simulink model "Car_23_Jan_test_2012b"  (R2012b)
settings: Solver=ode5  StartTime=0.0  StopTime=inf  FixedStep=sample_time  RelTol=1e-3
InitFcn:
  | sample_time=0.005;%0.004;%0.0025;%0.02;
  | sample_time_Vicon = 0.005;
  | DeltaT = 0.02;
  | g = 9.81;
  | H0 = g%0.3165;
  | Kl = 1;
  | 
  | Q6_mass = 0.84;
  | 
  | Q6_Omega_r = 1.5; %for horizon ref
  | Q6_Zeta_r = 0.5; %for horizon ref
  | Q6_Omega_r_h = 2;%for vertical ref
  | Q6_Zeta_r_h = 2; %for vertical ref
  | 
  | 
  | Q6_Omega = 1.5; %for horizon control
  | Q6_Zeta = 0.5; %for horizon control
  | Q6_Omega_h= 2; %for vertical control
  | Q6_Zeta_h = 0.7; %for vertical control
  | 
  | 
  | Q6_acc_max = 5;%horizontal max acc
  | Q6_acc_max_h = 3;%horizontal max acc
  | 
  | omega_circle = 72*pi/180;
  | omega_h = 0.1;%Ascending speed
  | PI = pi;
  | Circle_R = 2.5;
  | MAX_Height = -2;
undefined symbols (not defined in the file): DiscIntNeverNeededParam
libraries: X330_Control x5, dspswit3 x5, simulink x4
(part 2 of 2)

== matlab function Car_23_Jan_test_2012b/UAV 1/Trajectory Logic/trackbounded ==
  data: cpx input; cpy input; region output; cvx input; cvy input; newx output; newy output; newregion output; estsecond input; chkfinalx output; chkfinaly output; chknum output; directionflag output; distanceall output; limitspeed input
function [region,newx,newy,newregion,chkfinalx,chkfinaly,chknum,directionflag,distanceall]  = fcn(cpx,cpy,cvx,cvy,estsecond,limitspeed)
%#codegen
%cp = [cpy,cpx,0];
%cpest = [estrawy, estrawx,0];
%%database of check points
chk0x = -0.7975;
chk0y = 1.469;
chk1x = -1.008;
chk1y = 0.4326;
chk2x = -1.068;
chk2y = -0.6832;
chk3x = -0.5072;
chk3y = -1.342;
chk4x = 0.4105;
chk4y = -1.356;
chk5x = 1.225;
chk5y = -1.322;
chk6x = 1.733;
chk6y = -0.7022;
chk7x = 1.446;
chk7y = 0.6614;
chk8x = 1.136;
chk8y = 1.384;
chk9x = 0.3114;
chk9y = 1.798;
%%%%%%%%%%%%%%%%%%%%%%%%%%%%%%%%%%%%%%%%%%%%%%%%%%%%%%%%%%%
chk0 = [chk0y,chk0x,0];
chk1 = [chk1y,chk1x,0];
chk2 = [chk2y,chk2x,0];
chk3 = [chk3y,chk3x,0];
chk4 = [chk4y,chk4x,0];
chk5 = [chk5y,chk5x,0];
distance01 = sqrt((chk0y-chk1y)^2+(chk0x-chk1x)^2);
distance12 = sqrt((chk2y-chk1y)^2+(chk2x-chk1x)^2);
distance23 = sqrt((chk2y-chk3y)^2+(chk2x-chk3x)^2);
distance34 = sqrt((chk3y-chk4y)^2+(chk3x-chk4x)^2);
distance45 = sqrt((chk4y-chk5y)^2+(chk4x-chk5x)^2);
distance56 = sqrt((chk5y-chk6y)^2+(chk5x-chk6x)^2);
distance67 = sqrt((chk6y-chk7y)^2+(chk6x-chk7x)^2);
distance78 = sqrt((chk7y-chk8y)^2+(chk7x-chk8x)^2);
distance89 = sqrt((chk8y-chk9y)^2+(chk8x-chk9x)^2);
distance90 = sqrt((chk9y-chk0y)^2+(chk9x-chk0x)^2);
distanceall = distance01 + distance12 + distance23+distance34+distance45+distance56+distance67+distance78+distance89+distance90;
%%%%%%%%%%%%%%%%%%%%%%%%%%%%%%%%%%%%%%%%%%%%%%%%%%%%%%%%%%%%%%%%%%%%%%%%%%%%%%%%%%%%%%region selector
if(cpx>-2 && cpx<=-1 && cpy>1 && cpy<=2)
    region = 0;
elseif(cpx>-1 && cpx<=0 && cpy>1 && cpy<=2 )
    region = 1;
elseif(cpx>0 && cpx<=1 && cpy>1 && cpy<=2 )
    region = 2;
elseif(cpx>-2 && cpx<=-1 && cpy>0 &&cpy<=1)
    region = 3;
elseif(cpx>-1 && cpx<=0 && cpy>0 && cpy<=1)
    region = 4;
elseif(cpx>-2 && cpx<=-1 &&cpy>-1 && cpy<=0)
    region = 5;
elseif(cpx>-1 && cpx<=0 && cpy>-1 && cpy<=0)
    region = 6;
elseif(cpx>-2 && cpx<=-1 && cpy>-2 && cpy<=-1)
    region = 7;
elseif(cpx>-1 && cpx<=0 && cpy>-2 && cpy<=-1)
    region = 8;
elseif(cpx>0 && cpx<=1 && cpy>-2 && cpy<=-1)
    region = 9;
elseif(cpx>1 && cpx<=2 && cpy>-2 && cpy<=-1)
    region = 10;
elseif(cpx>0 && cpx<=1 && cpy>-1 && cpy<=0)
    region = 11;
elseif(cpx>1 && cpx<=2 && cpy>-1 && cpy<=0)
    region = 12;
elseif(cpx>1 && cpx<=2 && cpy>0 && cpy<=1)
    region = 13;
elseif(cpx>1 && cpx<=2 && cpy>1 && cpy<=2)
    region = 14;
elseif(cpx>0 && cpx<=1 && cpy>0 && cpy<=1)
    region = 15;
elseif(cpx>2 && cpx<=3 && cpy>-2 && cpy<=-1)
    region = 16;
elseif(cpx>1 && cpx<=2 && cpy>-3 && cpy<=-2)
    region = 17;
elseif(cpx>2 && cpx<=3 && cpy>-3 && cpy<=-2)
    region = 18;
elseif(cpx>0 && cpx<=1 && cpy>-3 && cpy<=-2)
    region = 19;
elseif(cpx>-1 && cpx<=0 && cpy>-3 && cpy<=-2)
    region = 20;
elseif(cpx>2 && cpx<=3 && cpy>-1 && cpy<=0)
    region = 21;
elseif(cpx>2 && cpx<=3 && cpy>0 && cpy<=1)
    region = 22;
elseif(cpx>1 && cpx<=2 && cpy>2 && cpy<=3)
    region = 23;
elseif(cpx>0 && cpx<=1 && cpy>2 && cpy<=3)
    region = 24;
elseif(cpx>-1 && cpx<=0 && cpy>2 && cpy<=3)
    region = 25;
else
    region = -1;
end
%%%%%%%%%%%%%%%%%%%%%%%%%%%%%%%%%%%%%%%%%%%%%%%%%%%%%%%%%%%%%%%%%%%%%%%%%%%%%%%%%%%%%%%%%%%%%%%%%%
if(region == 0 ||region==3||region==4)
    %%%%%%%%%%%%%%%%calculate point to line distance%%%%%%%%%%%
    %a = chk1 - chk0;
   % b = cp - chk0;
    %d = norm(cross(a,b)) / norm(a);
    angle = atan2((chk1x-chk0x),(chk1y-chk0y));
    samplex = chk0x;
    sampley = chk0y;
    zero = 1;

elseif(region == 5||region==6)
    %a = chk2 - chk1;
   % b = cp - chk1;
   % d = norm(cross(a,b)) / norm(a);
    angle = atan2((chk2x-chk1x),(chk2y-chk1y));
    zero = 1;
    samplex = chk1x;
    sampley = chk1y;
elseif(region == 7||region==8)
    %a = chk3 - chk2;
    %b = cp - chk2;
   % d = norm(cross(a,b)) / norm(a);
    angle = atan2((chk3x-chk2x),(chk3y-chk2y));
    zero = 1;
    samplex = chk2x;
    sampley = chk2y;
elseif(region == 9 || region==11||region==19||region==20)
   % a = chk4 - chk3;
   % b = cp - chk3;
    %d = norm(cross(a,b)) / norm(a);
    angle = atan2((chk4x-chk3x),(chk4y-chk3y));
    zero = 1;
      samplex = chk3x;
    sampley = chk3y;
elseif(region == 10 || region==17||region==18)
    %a = chk5 - chk4;
    %b = cp - chk4;
    %d = norm(cross(a,b)) / norm(a);
    angle = atan2((chk5x-chk4x),(chk5y-chk4y));
    zero = 1;
    samplex = chk4x;
    sampley = chk4y;
elseif(region == 12 || region==16||region==21)
    %a = chk6 - chk5;
    %b = cp - chk5;
    %d = norm(cross(a,b)) / norm(a);
    angle = atan2((chk6x-chk5x),(chk6y-chk5y));
    zero = 1;
    samplex = chk5x;
    sampley = chk5y;
elseif(region == 22 || region==13)
    %a = chk7 - chk6;
    %b = cp - chk6;
    %d = norm(cross(a,b)) / norm(a);
    angle = atan2((chk7x-chk6x),(chk7y-chk6y));
    zero = 1;
    samplex = chk6x;
    sampley = chk6y;
elseif(region == 14)
    %a = chk8 - chk7;
    %b = cp - chk7;
    %d = norm(cross(a,b)) / norm(a);
    angle = atan2((chk8x-chk7x),(chk8y-chk7y));
    zero = 1;
    samplex = chk7x;
    sampley = chk7y;
elseif(region == 2||region==23||region==24)
    %a = chk9 - chk8;
    %b = cp - chk8;
    %d = norm(cross(a,b)) / norm(a);
    angle = atan2((chk9x-chk8x),(chk9y-chk8y));
    zero = 1;
    samplex = chk8x;
    sampley = chk8y;
elseif(region == 25||region==1)
    %a = chk0 - chk9;
    %b = cp - chk9;
    %d = norm(cross(a,b)) / norm(a);
    angle = atan2((chk0x-chk9x),(chk0y-chk9y));
    zero = 1;
    samplex = chk9x;
    sampley = chk9y;
else
    %a = -1;
   % b = -1;
    %d = -1;
    angle = -1;%%% i know this is not correct i will add one more zero coefficient to cancel this case
    zero = 0;
    samplex = 0;
    sampley = 0;
end


%%%%%%%%%%%%%%%%%%%%%%%%%%%%%%%%%%%%%%%%%%%%%%%%%%%%%%%%%%%%%%%%%%%%%%%%%%%%%%%%%%%%%%%%%%%%%%%%%%
% %%calculate project point on the check point line
if(zero == 0)%%if out of boundary none of the region match
        newy = 100;
        newx = 100;
else   %%match the region

        if(angle == 0 ||angle == 180)
            newx  = samplex;
            newy = cpy;
        elseif(angle == 90 || angle == 270)
            newx = cpx;
            newy = sampley;
        else
         kk = -1/(tan(angle));
         m = cpx - kk*cpy ;
         k = tan(angle);
         newy = (samplex - k*sampley - m)/(kk - k);
         newx = kk*newy + m;
         end

end

if(newx>-2 && newx<=-1 && newy>1 && newy<=2)
    newregion = 0;
elseif(newx>-1 && newx<=0 && newy>1 && newy<=2 )
    newregion = 1;
elseif(newx>0 && newx<=1 && newy>1 && newy<=2 )
    newregion = 2;
elseif(newx>-2 && newx<=-1 && newy>0 &&newy<=1)
    newregion = 3;
elseif(newx>-1 && newx<=0 && newy>0 && newy<=1)
    newregion = 4;
elseif(newx>-2 && newx<=-1 &&newy>-1 && newy<=0)
    newregion = 5;
elseif(newx>-1 && newx<=0 && newy>-1 && newy<=0)
    newregion = 6;
elseif(newx>-2 && newx<=-1 && newy>-2 && newy<=-1)
    newregion = 7;
elseif(newx>-1 && newx<=0 && newy>-2 && newy<=-1)
    newregion = 8;
elseif(newx>0 && newx<=1 && newy>-2 && newy<=-1)
    newregion = 9;
elseif(newx>1 && newx<=2 && newy>-2 && newy<=-1)
    newregion = 10;
elseif(newx>0 && newx<=1 && newy>-1 && newy<=0)
    newregion = 11;
elseif(newx>1 && newx<=2 && newy>-1 && newy<=0)
    newregion = 12;
elseif(newx>1 && newx<=2 && newy>0 && newy<=1)
    newregion = 13;
elseif(newx>1 && newx<=2 && newy>1 && newy<=2)
    newregion = 14;
elseif(newx>0 && newx<=1 && newy>0 && newy<=1)
    newregion = 15;
elseif(newx>2 && newx<=3 && newy>-2 && newy<=-1)
    newregion = 16;
elseif(newx>1 && newx<=2 && newy>-3 && newy<=-2)
    newregion = 17;
elseif(newx>2 && newx<=3 && newy>-3 && newy<=-2)
    newregion = 18;
elseif(newx>0 && newx<=1 && newy>-3 && newy<=-2)
    newregion = 19;
elseif(newx>-1 && newx<=0 && newy>-3 && newy<=-2)
    newregion = 20;
elseif(newx>2 && newx<=3 && newy>-1 && newy<=0)
    newregion = 21;
elseif(newx>2 && newx<=3 && newy>0 && newy<=1)
    newregion = 22;
elseif(newx>1 && newx<=2 && newy>2 && newy<=3)
    newregion = 23;
elseif(newx>0 && newx<=1 && newy>2 && newy<=3)
    newregion = 24;
elseif(newx>-1 && newx<=0 && newy>2 && newy<=3)
    newregion = 25;
else
    newregion = -1;
end

%%%%%%%%%%%%%%%%%%%%%%%%%%%%%%%%%%%%%%%%%%%%%%%%%%%%%%%%%%%%%%%%%%%%%%%%%%%%
% if(posx>-2 && posx<=-1 && posy>1 && posy<=2)
%     posregion = 0;
% elseif(posx>-1 && posx<=0 && posy>1 && posy<=2 )
%     posregion = 1;
% elseif(posx>0 && posx<=1 && posy>1 && posy<=2 )
%     posregion = 2;
% elseif(posx>-2 && posx<=-1 && posy>0 &&posy<=1)
%     posregion = 3;
% elseif(posx>-1 && posx<=0 && posy>0 && posy<=1)
%     posregion = 4;
% elseif(posx>-2 && posx<=-1 &&posy>-1 && posy<=0)
%     posregion = 5;
% elseif(posx>-1 && posx<=0 && posy>-1 && posy<=0)
%     posregion = 6;
% elseif(posx>-2 && posx<=-1 && posy>-2 && posy<=-1)
%     posregion = 7;
% elseif(posx>-1 && posx<=0 && posy>-2 && posy<=-1)
%     posregion = 8;
% elseif(posx>0 && posx<=1 && posy>-2 && posy<=-1)
%     posregion = 9;
% elseif(posx>1 && posx<=2 && posy>-2 && posy<=-1)
%     posregion = 10;
% elseif(posx>0 && posx<=1 && posy>-1 && posy<=0)
%     posregion = 11;
% elseif(posx>1 && posx<=2 && posy>-1 && posy<=0)
%     posregion = 12;
% elseif(posx>1 && posx<=2 && posy>0 && posy<=1)
%     posregion = 13;
% elseif(posx>1 && posx<=2 && posy>1 && posy<=2)
%     posregion = 14;
% elseif(posx>0 && posx<=1 && posy>0 && posy<=1)
%     posregion = 15;
% elseif(posx>2 && posx<=3 && posy>-2 && posy<=-1)
%     posregion = 16;
% elseif(posx>1 && posx<=2 && posy>-3 && posy<=-2)
%     posregion = 17;
% elseif(posx>2 && posx<=3 && posy>-3 && posy<=-2)
%     posregion = 18;
% elseif(posx>0 && posx<=1 && posy>-3 && posy<=-2)
%     posregion = 19;
% elseif(posx>-1 && posx<=0 && posy>-3 && posy<=-2)
%     posregion = 20;
% elseif(posx>2 && posx<=3 && posy>-1 && posy<=0)
%     posregion = 21;
% elseif(posx>2 && posx<=3 && posy>0 && posy<=1)
%     posregion = 22;
% elseif(posx>1 && posx<=2 && posy>2 && posy<=3)
%     posregion = 23;
% elseif(posx>0 && posx<=1 && posy>2 && posy<=3)
%    posregion = 24;
% elseif(posx>-1 && posx<=0 && posy>2 && posy<=3)
%     posregion = 25;
% else
%     posregion = -1;
% end


%%%%%%%%%%%%%%%%%%%%%%%%%%%%%%%%%%%%%%%%%%%%%%%%%%%%%%%%%%%%%%%%%%%%%%%%%
velangle = atan2(cvx,cvy);
diffvelangletoangle = velangle - angle;
velproject = (cvx^2 + cvy^2)*cos(diffvelangletoangle);
estdistance = estsecond * velproject;
vxyM = sqrt(cvx^2 + cvy^2);
cosdiffvelangletoangle = cos(diffvelangletoangle);
if(vxyM < limitspeed)
    directionflag = 0;
    %frontbackflag = -1;
    %diffuavcartoangle = -9999;
else
if(cosdiffvelangletoangle>=0)
    directionflag = 1;
else
    directionflag = -1;
end
%uavcarvectorangle = atan2((posx-newx),(posy-newy));
%diffuavcartoangle = uavcarvectorangle - angle;
% cosdiffuavcartoangle = cos(diffuavcartoangle);
% if(cosdiffuavcartoangle>=0)
%     frontbackflag = 1;
% else
%     frontbackflag = 0;
% end
end
%if(directionflag == 1)
if(newregion == 0||newregion==3||newregion==4)
    newdistancetonext = sqrt((newy-chk1y)^2+(newx-chk1x)^2);
    if(estdistance < (newdistancetonext))
        chkfinalx = chk1x;
        chkfinaly = chk1y;
        chknum = 1;
    elseif(estdistance>=(newdistancetonext) && estdistance <((newdistancetonext) + distance12))
        chkfinalx = chk2x;
        chkfinaly = chk2y;
        chknum = 2;
    elseif(estdistance>=((newdistancetonext)+distance12)&&estdistance<((newdistancetonext)+distance12+distance23))
        chkfinalx = chk3x;
        chkfinaly = chk3y;
        chknum = 3;    
    else
        chkfinalx = chk3x;
        chkfinaly = chk3y;
        chknum = 3;
    end
elseif(newregion == 5||newregion==6)
    newdistancetonext = sqrt((newy-chk2y)^2+(newx-chk2x)^2);
    if(estdistance < (newdistancetonext))
        chkfinalx = chk2x;
        chkfinaly = chk2y;
        chknum = 2;
    elseif(estdistance >=(newdistancetonext)&&estdistance < ((newdistancetonext)+distance23))
        chkfinalx = chk3x;
        chkfinaly = chk3y;
        chknum = 3;
    elseif(estdistance >=((newdistancetonext)+distance23)&&estdistance < ((newdistancetonext)+distance23+distance34))
        chkfinalx = chk4x;
        chkfinaly = chk4y;
        chknum = 4;
    else
        chkfinalx = chk4x;
        chkfinaly = chk4y;
        chknum = 4;
    end
elseif(newregion == 7||newregion==8)
    newdistancetonext = sqrt((newy-chk3y)^2+(newx-chk3x)^2);
    if(estdistance < (newdistancetonext))
        chkfinalx = chk3x;
        chkfinaly = chk3y;
        chknum = 3;
    elseif((estdistance >= (newdistancetonext))&&estdistance<((newdistancetonext)+distance34))
        chkfinalx = chk4x;
        chkfinaly = chk4y;
        chknum = 4;
    elseif((estdistance >= (newdistancetonext)+distance34)&&estdistance<((newdistancetonext)+distance34+distance45))
        chkfinalx = chk5x;
        chkfinaly = chk5y;
        chknum = 5;
    else
        chkfinalx = chk5x;
        chkfinaly = chk5y;
        chknum = 5;
    end
elseif(newregion == 9 || newregion == 11||newregion==19||newregion==20)
    newdistancetonext = sqrt((newy-chk4y)^2+(newx-chk4x)^2);
    if(estdistance < (newdistancetonext))
        chkfinalx = chk4x;
        chkfinaly = chk4y;
        chknum = 4;
    elseif((estdistance >= (newdistancetonext))&&estdistance<((newdistancetonext)+distance45))
        chkfinalx = chk5x;
        chkfinaly = chk5y;
        chknum = 5;
    elseif((estdistance >= (newdistancetonext)+distance45)&&estdistance<((newdistancetonext)+distance45+distance56))
        chkfinalx = chk6x;
        chkfinaly = chk6y;
        chknum = 6;
    else
        chkfinalx = chk6x;
        chkfinaly = chk6y;
        chknum = 6;
    end
elseif(newregion == 10 || newregion == 17||newregion==18)
    newdistancetonext = sqrt((newy-chk5y)^2+(newx-chk5x)^2);
    if(estdistance < (newdistancetonext))
        chkfinalx = chk5x;
        chkfinaly = chk5y;
        chknum = 5;
    elseif((estdistance >= (newdistancetonext))&&estdistance<((newdistancetonext)+distance56))
        chkfinalx = chk6x;
        chkfinaly = chk6y;
        chknum = 6;
    elseif((estdistance >= (newdistancetonext)+distance56)&&estdistance<((newdistancetonext)+distance56+distance67))
        chkfinalx = chk7x;
        chkfinaly = chk7y;
        chknum = 7;
    else
        chkfinalx = chk7x;
        chkfinaly = chk7y;
        chknum = 7;
    end
elseif(newregion == 12 || newregion == 16||newregion==21)
    newdistancetonext = sqrt((newy-chk6y)^2+(newx-chk6x)^2);
    if(estdistance < (newdistancetonext))
        chkfinalx = chk6x;
        chkfinaly = chk6y;
        chknum = 6;
    elseif((estdistance >= (newdistancetonext))&&estdistance<((newdistancetonext)+distance67))
        chkfinalx = chk7x;
        chkfinaly = chk7y;
        chknum = 7;
    elseif((estdistance >= (newdistancetonext)+distance67)&&estdistance<((newdistancetonext)+distance67+distance78))
        chkfinalx = chk8x;
        chkfinaly = chk8y;
        chknum = 8;
    else
        chkfinalx = chk8x;
        chkfinaly = chk8y;
        chknum = 8;
    end
elseif(newregion == 13 || newregion == 22)
    newdistancetonext = sqrt((newy-chk7y)^2+(newx-chk7x)^2);
    if(estdistance < (newdistancetonext))
        chkfinalx = chk7x;
        chkfinaly = chk7y;
        chknum = 7;
    elseif((estdistance >= (newdistancetonext))&&estdistance<((newdistancetonext)+distance78))
        chkfinalx = chk8x;
        chkfinaly = chk8y;
        chknum = 8;
    elseif((estdistance >= (newdistancetonext)+distance78)&&estdistance<((newdistancetonext)+distance78+distance89))
        chkfinalx = chk9x;
        chkfinaly = chk9y;
        chknum = 9;
    else
        chkfinalx = chk9x;
        chkfinaly = chk9y;
        chknum = 9;
    end
elseif(newregion == 14)
    newdistancetonext = sqrt((newy-chk8y)^2+(newx-chk8x)^2);
    if(estdistance < (newdistancetonext))
        chkfinalx = chk8x;
        chkfinaly = chk8y;
        chknum = 8;
    elseif((estdistance >= (newdistancetonext))&&estdistance<((newdistancetonext)+distance89))
        chkfinalx = chk9x;
        chkfinaly = chk9y;
        chknum = 9;
    elseif((estdistance >= (newdistancetonext)+distance89)&&estdistance<((newdistancetonext)+distance89+distance90))
        chkfinalx = chk0x;
        chkfinaly = chk0y;
        chknum = 0;
    else
        chkfinalx = chk0x;
        chkfinaly = chk0y;
        chknum = 0;
    end
elseif(newregion == 2 || newregion == 23||newregion==24||newregion==15)
    newdistancetonext = sqrt((newy-chk9y)^2+(newx-chk9x)^2);
    if(estdistance < (newdistancetonext))
        chkfinalx = chk9x;
        chkfinaly = chk9y;
        chknum = 9;
    elseif((estdistance >= (newdistancetonext))&&estdistance<((newdistancetonext)+distance90))
        chkfinalx = chk0x;
        chkfinaly = chk0y;
        chknum = 0;
    else
        chkfinalx = chk0x;
        chkfinaly = chk0y;
        chknum = 0;
    end
elseif(newregion == 1 || newregion == 25)
    newdistancetonext = sqrt((newy-chk0y)^2+(newx-chk0x)^2);
    if(estdistance < (newdistancetonext))
        chkfinalx = chk0x;
        chkfinaly = chk0y;
        chknum = 0;
    else
        chkfinalx = chk0x;
        chkfinaly = chk0y;
        chknum = 0;
    end

else
    newdistancetonext = -1;
    chkfinalx = 0;
    chkfinaly = 0;
    chknum = -1;
    
end
% elseif(directionflag==-1)
%        if()
% else
%            
% end




%end
